simulink model "Simulink_Model_v12"  (R2020a)
settings: Solver=FixedStepAuto  StartTime=0.0  StopTime=150  FixedStep=1e-3  MaxStep=1e-2  RelTol=1e-3
PreLoadFcn:
  | addpath(genpath(pwd));
  | 
  | % ======================================================================= %
  | %% Physics Paramters
  | 
  | Physics_Param.gGravity        = 9.81;           % [m/s2]
  | Physics_Param.DAir            = 1.2;            % [kg/m3]
  | 
  | % ======================================================================= %
  | %% Tire Paramters
  | 
  | Tire_Param.muTire             = 1.75;           % [-]
  | 
  | Tire_Param.KTireLong          = 500;            % [rad^-1]
  | Tire_Param.KTireLat           = 1000;           % [rad^-1]
  | 
  | Tire_Param.CRollResistance    = 0.01;           % [-]
  | 
  | Tire_Param;
  | 
  | % ======================================================================= %
  | %% Motor Paramters
  | 
  | Motor_Param.PMotorMax         = 7.6*100;        % [W]
  | 
  | Motor_Param.nLimit            = 1000;           % [RPM]
  | 
  | Motor_Param.eDrivetrain       = 0.8*0.8*0.3;    % [-] %  \eta_i*\eta_d*correction_term
  | 
  | Motor_Param.rGearRatio1       = 3.3250;         % 84/48*38/20
  | Motor_Param.rGearRatio2       = 2.90;
  | 
  | % ======================================================================= %
  | %% Car Paramters
  | 
  | Car_Param.lCarWidth           = 0.2;            % [m]
  | Car_Param.hCarHeight          = 0.115;          % [m]
  | Car_Param.CCarDrag            = 0.3;            % [m]
  | 
  | Car_Param.lTrackWidth         = 0.165;          % [m]
  | Car_Param.lWheelbase          = 0.26;           % [m]
  | 
  | Car_Param.mWheel              = 0.03;           % [kg]
  | Car_Param.rWheel              = 0.03;           % [m]
  | Car_Param.IWheel              = 2.0760e-05;     % [kgm2] % 1/2*mWheel*(rWheel^2+0.022^2)
  | Car_Param.rWheelEffective     = 0.1885;         % [m]    % rWheel*2*pi
  | 
  | Car_Param.mCar                = 1.32;           % [kg]   % car mass
  | Car_Param.mCarSprung          = 1.198;          % [kg]   % mCar-4*mWheel
  | Car_Param.IzCar               = 0.0104;         % [kgm2] % 1/12*mCar*(lTrackWidth^2+lWheelbase^2)
  | 
  | Car_Param.hCenterGravity      = 0.02;           % [m]
  | 
  | Car_Param.hRollCenterF        = 0.01;           % [m]
  | Car_Param.hRollCenterR        = 0.01;           % [m]
  | 
  | Car_Param.KRollF              = 0.5;            % [N/m]
  | Car_Param.KRollR              = 0.5;            % [N/m]
  | 
  | Car_Param;
  | 
  | % ======================================================================= %
  | %% Track Select
  | 
  | % Track_Param.NTrack = 1;  % O-shape
  | % Track_Param.NTrack = 2;  % Oval-shape
  | 
  | Track_Param.NTrack = 5;  % Test track
  | % Track_Param.NTrack = 6;  % Test track
  | 
  | % Track_Param.NTrack = 10; % MCT
  | % Track_Param.NTrack = 11; % LMCC
  | 
  | % Track_Param.NTrack = 20; % AWS
  | 
  | run Track_Data\Track_Data.m
  | Track_Param.rTrajOpt = 0.009 %0.005;
  | 
  | % ======================================================================= %
  | %% Offline Trajectory Optimization
  | 
  | % run Trajectory_Optimizer.m
  | % Track_Param.xTrack=xTraj;
  | % Track_Param.yTrack=yTraj;
StopFcn:
  | Data1=out.CarPosition.Data;
  | 
  | figure(2)
  | cmap = colormap(jet);
  | s=scatter(Data1(:,1),Data1(:,2),0.1,Data1(:,4),'.');
  | c=colorbar;
  | ylabel(c,'v_{Car} (m/s)')
  | 
  | hold on
  | plot(Track_Param.xTrack,Track_Param.yTrack,'k')
  | plot(Track_Param.xRightSide',Track_Param.yRightSide','k--')
  | k=plot(Track_Param.xLeftSide' ,Track_Param.yLeftSide' ,'k--');
  | sf=plot(Track_Param.xStartLine,Track_Param.yStartLine,'k-.');
  | 
  | s.Annotation.LegendInformation.IconDisplayStyle = 'off';
  | k.Annotation.LegendInformation.IconDisplayStyle = 'off';
  | sf.Annotation.LegendInformation.IconDisplayStyle = 'off';
  | legend('Track centerline','Track limits')
  | axis off
  | text(0.5,-5,'S/F\rightarrow','HorizontalAlignment','center')
  | % title('Car position and velocity')
  | 
  | clear Data1 cmap s c k sf
libraries: simulink x8, dspfdesign x2
(part 1 of 2)
settings Model: Creator=arthu  LastModifiedBy=arthu
settings SolverCC: ZeroCrossAlgorithm=Adaptive
settings OptimizationCC: DefaultParameterBehavior=Inlined  EnhancedBackFolding=on  PassReuseOutputArgsAs=Individual arguments  ZeroExternalMemoryAtStartup=off  ZeroInternalMemoryAtStartup=off  OptimizeBlockOrder=speed  DifferentSizesBufferReuse=on  OptimizationCustomize=off  EfficientTunableParamExpr=on
settings DebuggingCC: ReadBeforeWriteMsg=DisableAll  WriteAfterWriteMsg=DisableAll  WriteAfterReadMsg=DisableAll  IgnoredZcDiagnostic=none  MultiTaskDSMMsg=none  ParameterTunabilityLossMsg=error
settings ModelReferenceCC: UpdateModelReferenceTargets=IfOutOfDate
settings SFSimCC: SFSimEcho=off  MATLABDynamicMemAlloc=off
settings RTWCC: SystemTargetFile=ert.tlc  TemplateMakefile=ert_default_tmf  BuildConfiguration=Faster Runs
settings CodeAppCC: ForceParamTrailComments=on  IgnoreCustomStorageClasses=off  OperatorAnnotations=on  SimulinkDataObjDesc=on  SFDataObjDesc=on  InsertBlockDesc=on
settings ERTTargetCC: TargetLangStandard=C99 (ISO)  GenerateSampleERTMain=on  InlinedParameterPlacement=NonHierarchical  ERTCustomFileTemplate=example_file_process.tlc

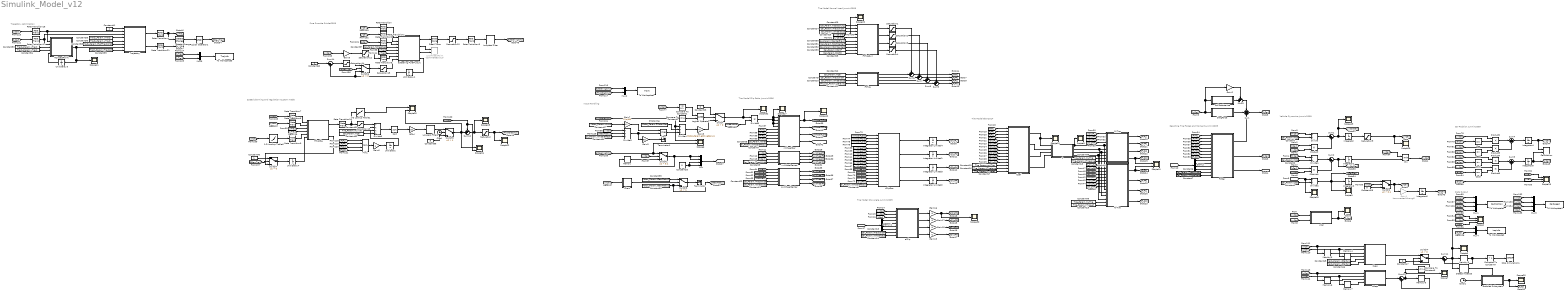
== system Simulink_Model_v12 ==
  note: Trajectory optimization
  note: Speed planning and regulation
      |
      | Custom made
  note: Pure Pursuite
      |
      | Snider2009
  note: Input Handling
  note: Tire Model
      | Slip Ratio
      |
      | Junmin2006
  note: Tire Model
      | Slip Angle
      |
      | Junmin2009
  note: Tire Model
      | Normal Load
      |
      | Junmin2009
  note: Tire Model
      |
      | Bian2014
  note: Resulting Tire Forces and Moment
      |
      | Junmin2009
  note: Vehicle Dynamics
      |
      | Junmin2009
  note: Data Output
  note: Car Position
      |
      | Junmin2009
  1-D Lookup Table1 : Lookup_n-D  NumberOfTableDimensions=1  BreakpointsForDimension1=[0,0.04,0.1,0.2,0.3,0.5]*1  Table=[20,10,9,6,5,4]  ExtrapMethod=Clip  InternalRulePriority=Speed  RndMeth=Simplest  InputSameDT=on
  1-D Lookup Table6 : Lookup_n-D  NumberOfTableDimensions=1  BreakpointsForDimension1=[7.5,10,15,20]  Table=[5,10,25,40]  ExtrapMethod=Clip  InternalRulePriority=Speed  OutDataTypeStr=Inherit: Inherit via back propagation  RndMeth=Simplest  InputSameDT=on
  CarPosition : simulink/Sinks/XY Graph  xmin=min(Track_Param.xTrack)-10  xmax=max(Track_Param.xTrack)+10  ymin=min(Track_Param.yTrack)-10  ymax=max(Track_Param.yTrack)+10  st=-1
  Chart : Stateflow chart  TreatAsAtomicUnit=on
  Clock : Clock
  Clock1 : Clock
  Coef : MATLAB Function  TreatAsAtomicUnit=on
  Compare To Constant1 : simulink/Logic and Bit Operations/Compare To Constant  relop=<=  const=0.1  OutDataTypeStr=boolean
  Compare To Constant2 : simulink/Logic and Bit Operations/Compare To Constant  relop=<=  const=0  OutDataTypeStr=boolean
  Compare To Constant3 : simulink/Logic and Bit Operations/Compare To Constant  relop=>=  const=1  OutDataTypeStr=boolean
  Compare To Constant4 : simulink/Logic and Bit Operations/Compare To Constant  relop=>  const=4  OutDataTypeStr=boolean
  Constant{,2,12,52} (4 alike) : Constant  Value=Car_Param.mCar
  Constant1 : Constant  Value=Car_Param.IzCar
  Constant{7,10,14,21,26,37} (6 alike) : Constant  Value=Car_Param.lWheelbase
  Constant11 : Constant  Value=Physics_Param.gGravity
  Constant{3,6,9,13,22,24} (6 alike) : Constant  Value=Car_Param.lTrackWidth
  Constant{15,48..49,51} (4 alike) : Constant  Value=Tire_Param.muTire
  Constant16 : Constant  Value=Tire_Param.KTireLong
  Constant17 : Constant  Value=Tire_Param.KTireLat
  Constant18 : Constant  Value=Tire_Param.KTireLong
  Constant19 : Constant  Value=Tire_Param.KTireLat
  Constant{20,23,28,47} (4 alike) : Constant  Value=0
  Constant25 : Constant  Value=Car_Param.KRollR
  Constant27 : Constant  Value=Motor_Param.nLimit  SampleTime=-1
  Constant29 : Constant  Value=Car_Param.mCarSprung
  Constant30 : Constant  Value=Car_Param.hCenterGravity
  Constant31 : Constant  Value=Car_Param.hRollCenterF
  Constant32 : Constant  Value=Car_Param.hRollCenterR
  Constant33 : Constant  Value=Car_Param.KRollF
  Constant34 : Constant  Value=Car_Param.rWheelEffective  SampleTime=-1
  Constant35 : Constant  Value=Motor_Param.rGearRatio2  SampleTime=-1
  Constant36 : Constant  Value=5
  Constant39 : Constant  Value=Track_Param.rTrajOpt
  Constant4 : Constant  Value=Car_Param.rWheelEffective  SampleTime=-1
  Constant40 : Constant
  Constant41 : Constant  OutDataTypeStr=boolean
  Constant45 : Constant  Value=Track_Param.xStartLine
  Constant46 : Constant  Value=Track_Param.yStartLine
  Constant5 : Constant  Value=Car_Param.IWheel  SampleTime=-1
  Constant50 : Constant  Value=Motor_Param.rGearRatio1  SampleTime=-1
  Constant53 : Constant  Value=Track_Param.xTrack
  Constant54 : Constant  Value=Track_Param.yTrack
  Constant55 : Constant  Value=Track_Param.xTrack
  Constant56 : Constant  Value=Track_Param.yTrack
  Constant58 : Constant  Value=Track_Param.lHalfTrackWidth
  Constant60 : Constant
  Constant8 : Constant  Value=Car_Param.rWheelEffective  SampleTime=-1
  Cos : Trigonometry  Operator=cos
  Cos1 : Trigonometry
  Cos2 : Trigonometry
  Cos3 : Trigonometry  Operator=cos
  Dead Zone : DeadZone  LowerValue=-0.5*pi/180  UpperValue=0.5*pi/180  SaturateOnIntegerOverflow=on
  Demux : Demux
  Demux1 : Demux
  Detect Change : simulink/Logic and Bit Operations/Detect Change  vinit=0  OutDataTypeStr=boolean
  Detect Increase : simulink/Logic and Bit Operations/Detect Increase  vinit=0.0  OutDataTypeStr=boolean
  Divide : Product  Inputs=*/
  Divide1 : Product  Inputs=*/
  Divide2 : Product  Inputs=*/
  Divide3 : Product  Inputs=**/
  Divide4 : Product  Inputs=**/
  Divide5 : Product  Inputs=/**/
  Divide6 : Product  Inputs=**
  DragForce : Subsystem
  Enabled Subsystem : Subsystem  TreatAsAtomicUnit=on
  FMCar : MATLAB Function  TreatAsAtomicUnit=on
  FxTire : MATLAB Function  TreatAsAtomicUnit=on
  FyTire : MATLAB Function  TreatAsAtomicUnit=on
  FzTire : MATLAB Function  TreatAsAtomicUnit=on
  FzTireDyn : MATLAB Function  TreatAsAtomicUnit=on
  Gain1 : Gain  Commented=through  Gain=1/10
  Gain{16..19} (4 alike) : Gain  Gain=-1
  Gain2 : Gain  Gain=0.05
  Gain3 : Gain  Gain=60
  Gain5 : Gain  Gain=0.25
  Gain6 : Gain  Gain=4
  Gain7 : Gain  Gain=2*pi/60
  Gain8 : Gain  Gain=Motor_Param.eDrivetrain/4
  Integrator{,2,4..6} (5 alike) : Integrator
  Integrator Limited{1..4} (4 alike) : Integrator  LimitOutput=on  UpperSaturationLimit=10*pi/180  LowerSaturationLimit=-10*pi/180
  Integrator1 : Integrator  LimitOutput=on  UpperSaturationLimit=1  LowerSaturationLimit=-1
  Logical Operator : Logic  AllPortsSameDT=off  OutDataTypeStr=boolean
  Logical Operator1 : Logic  Inputs=1  AllPortsSameDT=off  OutDataTypeStr=boolean
  LookAheadPoint : simulink/Sinks/XY Graph  Commented=on  xmin=min(Track_Param.xTrack)-10  xmax=max(Track_Param.xTrack)+10  ymin=min(Track_Param.yTrack)-10  ymax=max(Track_Param.yTrack)+10  st=-1
  Lowpass Filter : dspfdesign/Lowpass Filter  FilterType=FIR  DesignForMinimumOrder=on  FilterOrder=50  PassbandFrequency=50  StopbandFrequency=100  PassbandRipple=0.1  StopbandAttenuation=50  InheritSampleRate=off  SampleRate=1000  SimulateUsing=Interpreted execution  roundingMode=Floor  coeffsDataTypeStr=fixdt(1,16)
  Lowpass Filter1 : dspfdesign/Lowpass Filter  FilterType=FIR  DesignForMinimumOrder=on  FilterOrder=50  PassbandFrequency=2  StopbandFrequency=10  PassbandRipple=0.1  StopbandAttenuation=50  InheritSampleRate=off  SampleRate=1000  SimulateUsing=Interpreted execution  roundingMode=Floor  coeffsDataTypeStr=fixdt(1,16)
  Max : MinMax  Function=max  Inputs=2
  Memory{,3..4,6..8} (6 alike) : Memory
  Memory5 : Memory  InitialCondition=1
  Min : MinMax  Inputs=2
  Min1 : MinMax  Inputs=4
  Mux : Mux
  Mux1 : Mux
  Mux2 : Mux  Inputs=2
  Mux3 : Mux  Inputs=2
  Mux4 : Mux  Inputs=2
  Mux5 : Mux
  NClosestPoint : MATLAB Function  TreatAsAtomicUnit=on
  NLap : MATLAB Function  TreatAsAtomicUnit=on
  PMotorMax : Constant  Value=Motor_Param.PMotorMax  SampleTime=-1
  Product{,1..5} (6 alike) : Product
  Rate Transition{,1..2,4..5,7..9,21} (9 alike) : RateTransition  OutPortSampleTime=0.01
  Rate Transition10 : RateTransition  OutPortSampleTime=0.001
  Rate Transition16 : RateTransition  OutPortSampleTime=0.1
  Rate Transition17 : RateTransition  OutPortSampleTime=0.1
  Rate Transition3 : RateTransition  OutPortSampleTime=0.001
  RollResistance : Subsystem
  Saturation : Saturate  UpperLimit=1  LowerLimit=-1
  Saturation{1..4} (4 alike) : Saturate  UpperLimit=Car_Param.mCar*Physics_Param.gGravity  LowerLimit=-Car_Param.mCar*Physics_Param.gGravity/4
  Saturation10 : Saturate  UpperLimit=26*pi/180  LowerLimit=-26*pi/180
  Saturation12 : Saturate  UpperLimit=5  LowerLimit=1
  Saturation13 : Saturate  UpperLimit=inf  LowerLimit=0.01
  Saturation14 : Saturate  UpperLimit=100  LowerLimit=1
  Saturation15 : Saturate  UpperLimit=100  LowerLimit=1
  Saturation9 : Saturate  UpperLimit=inf  LowerLimit=0
  Scope{,3,5,7,9,11..13,16..17,19..20,22,25,28..30,32} (18 alike) : Scope
  Scope{6,10,26,34} (4 alike) : Scope  NumInputPorts=2
  Scope15 : Scope  NumInputPorts=3
  Scope2 : Scope  NumInputPorts=3
  Sqrt : Sqrt  SaturateOnIntegerOverflow=on
  Stop Simulation1 : Stop
  Sum : Sum  Inputs=--+
  Sum{1,5,11,13} (4 alike) : Sum  Inputs=|++
  Sum12 : Sum  Inputs=-+|
  Sum14 : Sum  Inputs=|-+
  Sum2 : Sum  Inputs=|+-
  Sum{3,6..9} (5 alike) : Sum  Inputs=++|
  Sum4 : Sum  Inputs=|+-
  Switch{,4,6..7} (4 alike) : Switch  Criteria=u2 > Threshold
  Switch1 : Switch  Criteria=u2 > Threshold  Threshold=0.1
  Switch2 : Switch  Criteria=u2 > Threshold  Threshold=0.1
  Switch5 : Switch  Criteria=u2 > Threshold  Threshold=1
  Switch8 : Switch  Criteria=u2 > Threshold  Threshold=1
  Terminator : Terminator
  Terminator1 : Terminator
  To Workspace : ToWorkspace  VariableName=CarPosition  SaveFormat=Timeseries  SampleTime=-1
  To Workspace1 : ToWorkspace  VariableName=Input  SaveFormat=Timeseries  SampleTime=-1
  To Workspace2 : ToWorkspace  VariableName=LapInfo  SaveFormat=Timeseries  SampleTime=-1
  To Workspace3 : ToWorkspace  VariableName=TrajInfo  SaveFormat=Timeseries  SampleTime=-1
  To Workspace4 : ToWorkspace  VariableName=CarSpeed  SaveFormat=Timeseries  SampleTime=-1
  Trajectory : MATLAB Function  TreatAsAtomicUnit=on
  Unit Delay : UnitDelay  SampleTime=0.001  HasFrameUpgradeWarning=on
  Unit Delay1 : UnitDelay  InitialCondition=1  SampleTime=-1  HasFrameUpgradeWarning=on
  Unit Delay3 : UnitDelay  InitialCondition=1  SampleTime=-1  HasFrameUpgradeWarning=on
  Unit Delay4 : UnitDelay  InitialCondition=1  SampleTime=-1  HasFrameUpgradeWarning=on
  \eta_v : Gain  Gain=0.8
  aSlip : MATLAB Function  TreatAsAtomicUnit=on
  aSteering PurePursuit : MATLAB Function  TreatAsAtomicUnit=on
  axWheelCenter : MATLAB Function  TreatAsAtomicUnit=on
  f : MATLAB Function  TreatAsAtomicUnit=on
  nWheelDer : MATLAB Function  TreatAsAtomicUnit=on
  rSlipDer : MATLAB Function  TreatAsAtomicUnit=on
  rThrottle : MATLAB Function  TreatAsAtomicUnit=on
  sStep : MATLAB Function  TreatAsAtomicUnit=on
  vCar : MATLAB Function  TreatAsAtomicUnit=on
  vxWheelCenter : MATLAB Function  TreatAsAtomicUnit=on
  wires:
  [FxCar] -> Divide/1
  Constant/1 -> Divide/2
  Divide/1 -> Sum1/1
  [rCar] -> Product/1
  [vyCar] -> Product/2
  Product/1 -> Sum1/2
  Sum1/1 -> Scope19/1, [vxCarDer], Integrator/1
  Integrator/1 -> Saturation9/1
  [vxCar] -> Product1/2
  [rCar] -> Product1/1
  Constant2/1 -> Divide1/2
  [FyCar] -> Divide1/1
  Divide1/1 -> Sum2/1
  Product1/1 -> Sum2/2
  Sum2/1 -> [vyCarDer], Integrator1/1
  Demux1/1 -> aSlip/4(aSteerFL)
  FMCar/1(FxCar) -> Sum/3
  Sum/1 -> [FxCar]
  DragForce/1(FDrag) -> Sum/2
  [vxCar] -> vCar/1(vxCar)
  [vyCar] -> vCar/2(vyCar)
  vCar/1(vCar) -> [vCar], Scope/1  "vCar"
  [vCar] -> Gain2/1, RollResistance/1(vCar), DragForce/1(vCar)
  [aSteer] -> Demux/1
  Demux/1 -> FMCar/9(aSteerFL)
  Demux/4 -> FMCar/12(aSteerRR)
  Demux/2 -> FMCar/10(aSteerFR)
  Demux/3 -> FMCar/11(aSteerRL)
  Constant6/1 -> FMCar/13(lTrackWidth)
  Constant7/1 -> FMCar/14(lWheelbase)
  Constant3/1 -> vxWheelCenter/4(lTrackWidth)
  [rCar] -> vxWheelCenter/3(rCar)
  [vyCar] -> vxWheelCenter/2(vyCar)
  [vxCar] -> vxWheelCenter/1(vxCar)
  Constant8/1 -> rSlipDer/17(rWheelEffective)
  FzTire/1(FzFL) -> Sum6/2  "FzFL"
  FzTire/2(FzFR) -> Sum7/2  "FzFR"
  FzTire/3(FzRL) -> Sum8/2  "FzRL"
  FzTire/4(FzRR) -> Sum9/2  "FzRR"
  Constant12/1 -> FzTire/1(mCar)
  Constant9/1 -> FzTire/2(lTrackWidth)
  Constant10/1 -> FzTire/3(lWheelbase)
  Constant11/1 -> FzTire/4(gGravity)
  [rCar] -> aSlip/3(rCar)
  [vxCar] -> aSlip/1(VxCar)
  [vyCar] -> aSlip/2(VyCar)
  [aSteer] -> Demux1/1
  Demux1/2 -> aSlip/5(aSteerFR)
  Demux1/3 -> aSlip/6(aSteerRL)
  Demux1/4 -> aSlip/7(aSteerRR)
  Constant13/1 -> aSlip/8(lTrackWidth)
  Constant14/1 -> aSlip/9(lWheelbase)
  [FzFL] -> Coef/1(FzFL)
  [FzFR] -> Coef/2(FzFR)
  [FzRL] -> Coef/3(FzRL)
  [FzRR] -> Coef/4(FzRR)
  aSlip/1(aSlipFL) -> Gain16/1  "aSlipFL"
  aSlip/2(aSlipFR) -> Gain17/1  "aSlipFR"
  aSlip/3(aSlipRL) -> Gain18/1  "aSlipRL"
  aSlip/4(aSlipRR) -> Gain19/1  "aSlipRR"
  Constant15/1 -> Coef/13(muTire)
  Constant16/1 -> Coef/14(KTireLong)
  Constant17/1 -> Coef/15(KTireLat)
  [rSlipFR] -> Coef/6(rSlipFR)
  [rSlipFL] -> Coef/5(rSlipFL)
  [rSlipRL] -> Coef/7(rSlipRL)
  [rSlipRR] -> Coef/8(rSlipRR)
  [aSlipFL] -> Coef/9(aSlipFL)
  [aSlipFR] -> Coef/10(aSlipFR)
  [aSlipRL] -> Coef/11(aSlipRL)
  [aSlipRR] -> Coef/12(aSlipRR)
  Coef/1(CoefFL) -> Scope13/1, f/1(CoefFL)
  Coef/2(CoefFR) -> f/2(CoefFR)
  Coef/3(CoefRL) -> f/3(CoefRL)
  Coef/4(CoefRR) -> f/4(CoefRR)
  f/1(fCoefFL) -> FyTire/9(fCoefFL), FxTire/5(fCoefFL), Scope9/1
  f/2(fCoefFR) -> FyTire/10(fCoefFR), FxTire/6(fCoefFR)
  f/3(fCoefRL) -> FyTire/11(fCoefRL), FxTire/7(fCoefRL)
  f/4(fCoefRR) -> FxTire/8(fCoefRR), FyTire/12(fCoefRR)
  [rSlipFL] -> FxTire/1(rSlipFL)
  [rSlipFR] -> FxTire/2(rSlipFR)
  [rSlipRL] -> FxTire/3(rSlipRL)
  [rSlipRR] -> FxTire/4(rSlipRR)
  Constant18/1 -> FxTire/10(KTireLong)
  [FxFL] -> FMCar/1(FxFL)
  [FxFR] -> FMCar/2(FxFR)
  [FxRL] -> FMCar/3(FxRL)
  [FxRR] -> FMCar/4(FxRR)
  [rSlipFL] -> FyTire/5(rSlipFL)
  [rSlipFR] -> FyTire/6(rSlipFR)
  [rSlipRL] -> FyTire/7(rSlipRL)
  [rSlipRR] -> FyTire/8(rSlipRR)
  Constant19/1 -> FyTire/14(KTireLat)
  [aSlipFL] -> FyTire/1(aSlipFL)
  [aSlipFR] -> FyTire/2(aSlipFR)
  [aSlipRL] -> FyTire/3(aSlipRL)
  [aSlipRR] -> FyTire/4(aSlipRR)
  FyTire/1(FyFL) -> Scope10/2, [FyFL]
  FyTire/2(FyFR) -> [FyFR]
  FyTire/3(FyRL) -> [FyRL]
  FyTire/4(FyRR) -> [FyRR]
  [FyFL] -> FMCar/5(FyFL)
  [FyFR] -> FMCar/6(FyFR)
  [FyRL] -> FMCar/7(FyRL)
  [FyRR] -> FMCar/8(FyRR)
  Gain17/1 -> [aSlipFR]
  Gain18/1 -> [aSlipRL]
  Gain19/1 -> [aSlipRR]
  Mux/1 -> [aSteer]
  FxTire/1(FxFL) -> [FxFL]
  FxTire/2(FxFR) -> [FxFR]
  FxTire/3(FxRL) -> [FxRL]
  FxTire/4(FxRR) -> [FxRR], Scope10/1
  [vxCar] -> Scope2/1  "vxCar"
  [vyCar] -> Scope2/2  "vyCar"
  [rCar] -> Scope2/3  "rCar"
  Integrator Limited4/1 -> [rSlipFL]
  Integrator Limited1/1 -> [rSlipFR]
  Integrator Limited3/1 -> [rSlipRL]
  Integrator Limited2/1 -> [rSlipRR]
  Constant20/1 -> Mux/3, Mux/4
  Switch1/1 -> Memory/1, Mux/2, Mux/1
  vxWheelCenter/1(vxWheelFL) -> [vxWheelFL]
  vxWheelCenter/2(vxWheelFR) -> [vxWheelFR]
  vxWheelCenter/3(vxWheelRL) -> [vxWheelRL]
  vxWheelCenter/4(vxWheelRR) -> [vxWheelRR]
  [vxWheelRR] -> rSlipDer/8(vxWheelRR)
  [vxWheelRL] -> rSlipDer/7(vxWheelRL)
  [vxWheelFR] -> rSlipDer/6(vxWheelFR)
  [vxWheelFL] -> rSlipDer/5(vxWheelFL)
  [FxFL] -> nWheelDer/5(FxFL)
  [FxFR] -> nWheelDer/6(FxFR)
  [FxRL] -> nWheelDer/7(FxRL)
  [FxRR] -> nWheelDer/8(FxRR)
  Constant4/1 -> nWheelDer/10(rWheelEffective)
  Constant5/1 -> nWheelDer/9(IWheel)
  [rCar] -> axWheelCenter/1(rCar)
  [vxCarDer] -> axWheelCenter/2(vxCarDer)
  [vyCarDer] -> axWheelCenter/3(vyCarDer)
  [rCarDer] -> axWheelCenter/4(rCarDer)
  Constant21/1 -> axWheelCenter/6(lWheelbase)
  Constant22/1 -> axWheelCenter/5(lTrackWidth)
  axWheelCenter/1(axWheelFL) -> [axWheelFL]
  axWheelCenter/2(axWheelFR) -> [axWheelFR]
  axWheelCenter/3(axWheelRL) -> [axWheelRL]
  axWheelCenter/4(axWheelRR) -> [axWheelRR]
  [axWheelFR] -> rSlipDer/10(axWheelFR)
  [axWheelFL] -> rSlipDer/9(axWheelFL)
  [axWheelRL] -> rSlipDer/11(axWheelRL)
  [axWheelRR] -> rSlipDer/12(axWheelRR)
  [rSlipFL] -> rSlipDer/13(rSlipFL)
  [rSlipFR] -> rSlipDer/14(rSlipFR)
  [rSlipRL] -> rSlipDer/15(rSlipRL)
  [rSlipRR] -> rSlipDer/16(rSlipRR)
  Divide6/1 -> nWheelDer/1(MWheelFL), Scope17/1, nWheelDer/2(MWheelFR), nWheelDer/3(MWheelRL), nWheelDer/4(MWheelRR)  "MWheel"
  nWheelDer/1(nWheelFLDer) -> Scope12/1, [nWheelFLDer]
  nWheelDer/2(nWheelFRDer) -> [nWheelFRDer]
  nWheelDer/4(nWheelRRDer) -> [nWheelRRDer]
  nWheelDer/3(nWheelRLDer) -> [nWheelRLDer]
  [nWheelFLDer] -> rSlipDer/1(nWheelFLDer)
  [nWheelFRDer] -> rSlipDer/2(nWheelFRDer)
  [nWheelRLDer] -> rSlipDer/3(nWheelRLDer)
  [nWheelRRDer] -> rSlipDer/4(nWheelRRDer)
  Logical Operator/1 -> Switch/2
  [vCar] -> Compare To Constant1/1
  Compare To Constant1/1 -> Logical Operator/1
  Constant23/1 -> Switch/1
  [MzCar] -> Scope16/1, Divide2/1
  Sum4/1 -> Integrator4/1
  [vyCar] -> Product5/1
  Product5/1 -> Sum5/2
  Cos2/1 -> Product4/2
  Cos3/1 -> Product5/2
  [vxCar] -> Product4/1
  Product4/1 -> Sum5/1
  [aCar] -> Scope15/3  "aCar"
  [vyCar] -> Product3/1
  Cos1/1 -> Product3/2
  [aCar] -> Cos2/1
  Sum5/1 -> Integrator5/1
  [vxCar] -> Product2/1
  Cos/1 -> Product2/2
  [aCar] -> Cos3/1
  [aCar] -> Cos/1
  Product3/1 -> Sum4/2
  [aCar] -> Cos1/1
  Product2/1 -> Sum4/1
  Integrator6/1 -> [aCar]
  Integrator4/1 -> CarPosition/1, [xCar]  "xCar"
  Switch2/1 -> Gain1/1, [rCar]
  FMCar/2(FyCar) -> [FyCar]
  [yCar] -> Mux1/2
  [xCar] -> Mux1/1
  Mux1/1 -> To Workspace/1
  [vCar] -> Mux1/4
  Constant26/1 -> FzTireDyn/3(lWheelbase)
  Constant33/1 -> FzTireDyn/9(KRollF)
  Constant29/1 -> FzTireDyn/1(mCarSprung)
  Constant25/1 -> FzTireDyn/10(KRollR)
  Constant30/1 -> FzTireDyn/6(hCentrerGravity)
  Constant24/1 -> FzTireDyn/2(lTrackWidth)
  Constant32/1 -> FzTireDyn/8(hRollCenterR)
  Constant31/1 -> FzTireDyn/7(hRollCenterF)
  [vxCarDer] -> Scope20/1, FzTireDyn/4(axCar)
  [vyCarDer] -> FzTireDyn/5(ayCar)
  Sum9/1 -> [FzRR]  "FzRR"
  Sum8/1 -> [FzRL]  "FzRL"
  Sum7/1 -> [FzFR]  "FzFR"
  Sum6/1 -> [FzFL]  "FzFL"
  Integrator5/1 -> CarPosition/2, [yCar]  "yCar"
  [xCar] -> Scope15/1
  [yCar] -> Scope15/2
  FzTireDyn/4(FzRR) -> Saturation4/1
  FzTireDyn/3(FzRL) -> Saturation3/1
  FzTireDyn/2(FzFR) -> Saturation2/1
  FzTireDyn/1(FzFL) -> Saturation1/1
  Sum3/1 -> Sum/1
  [vxCar] -> Min/1
  Constant28/1 -> Switch2/3
  [vxCar] -> Switch2/2
  Compare To Constant2/1 -> Logical Operator/2
  [vxCar] -> Divide3/1
  Constant34/1 -> Divide3/3
  Divide3/1 -> Gain3/1, Max/2  "nMotor tr/s"
  PMotorMax/1 -> Divide4/2
  Divide4/1 -> Gain8/1
  Min/1 -> [vyCar]
  Constant27/1 -> Gain7/1
  Max/1 -> Divide4/3
  [vxCar] -> Switch1/2
  Memory/1 -> Switch1/3
  Constant1/1 -> Divide2/2
  Saturation9/1 -> Scope29/1, [vxCar]
  Integrator1/1 -> Min/2
  Integrator2/1 -> Switch2/1
  Gain1/1 -> Integrator6/1
  Divide2/1 -> [rCarDer], Scope3/1, Integrator2/1
  RollResistance/1(FRollResistance) -> Sum3/2
  Gain2/1 -> Sum3/1
  [xCar] -> Rate Transition/1
  [yCar] -> Rate Transition1/1
  [aCar] -> Rate Transition2/1
  Constant37/1 -> aSteering PurePursuit/4(lWheelBase)
  Dead Zone/1 -> Saturation10/1
  Rate Transition/1 -> aSteering PurePursuit/1(xCar)
  Rate Transition1/1 -> aSteering PurePursuit/2(yCar)
  Rate Transition2/1 -> aSteering PurePursuit/3(aCar)
  aSteering PurePursuit/3(yLookAheadPoint) -> LookAheadPoint/2
  aSteering PurePursuit/2(xLookAheadPoint) -> LookAheadPoint/1
  [rThrottleCmd] -> Scope6/1, Divide4/1, Compare To Constant2/1
  [aSteeringCmd] -> Scope6/2, Switch1/1
  [vxCar] -> Scope34/2, Sum12/1
  Rate Transition5/1 -> aSteering PurePursuit/7(sLookAhead)
  Rate Transition8/1 -> rThrottle/2(yCar)
  Rate Transition7/1 -> rThrottle/1(xCar)
  [yCar] -> Rate Transition8/1
  [xCar] -> Rate Transition7/1
  rThrottle/1(KMax) -> Rate Transition10/1
  [vxCar] -> 1-D Lookup Table6/1
  Rate Transition9/1 -> rThrottle/5(sAnticipation)
  Saturation1/1 -> Sum6/1
  Saturation2/1 -> Sum7/1
  Saturation3/1 -> Sum8/1
  Saturation4/1 -> Sum9/1
  Saturation/1 -> Scope22/1, [rThrottleCmd]
  \eta_v/1 -> Lowpass Filter1/1
  Constant45/1 -> NLap/5(xStartLine)
  Constant46/1 -> NLap/6(yStartLine)
  [xCar] -> Memory3/1, NLap/1(xCar)
  [yCar] -> Memory4/1, NLap/2(yCar)
  Memory3/1 -> NLap/3(xCarPrev)
  Memory4/1 -> NLap/4(yCarPrev)
  NLap/1(BNewLap) -> Switch4/1
  Sum11/1 -> Mux4/1, Scope5/1, Detect Increase/1, Memory5/1  "NLap"
  Memory5/1 -> Compare To Constant4/1, Sum11/2
  Memory6/1 -> sStep/3(xCarPrev)
  Memory7/1 -> sStep/4(yCarPrev)
  [yCar] -> Memory7/1, sStep/2(yCar)
  [xCar] -> Memory6/1, sStep/1(xCar)
  Memory8/1 -> Sum13/2
  Sum13/1 -> Memory8/1, Scope7/1, Compare To Constant3/1  "sCovered"
  sStep/1(sStep) -> Sum13/1
  Compare To Constant3/1 -> Switch4/2
  Switch4/1 -> Sum11/1
  Constant47/1 -> Switch4/3
  Lowpass Filter/1 -> [aSteeringCmd]
  aSteering PurePursuit/1(aSteeringCmd) -> Dead Zone/1
  [aSteeringCmd] -> Mux2/1
  Mux2/1 -> To Workspace1/1
  [rThrottleCmd] -> Mux2/2
  [FzFL] -> Min1/1
  [FzFR] -> Min1/2
  [FzRL] -> Min1/3
  [FzRR] -> Min1/4
  Divide5/1 -> Sqrt/1
  Sqrt/1 -> \eta_v/1
  Constant51/1 -> Divide5/3
  Constant52/1 -> Divide5/4
  Saturation13/1 -> Divide5/1
  Min1/1 -> Gain6/1
  Gain6/1 -> Unit Delay/1
  Unit Delay/1 -> Divide5/2
  Gain7/1 -> Max/1
  Gain8/1 -> Switch/3
  Saturation10/1 -> Rate Transition3/1
  Rate Transition3/1 -> Lowpass Filter/1
  Clock/1 -> Switch5/2
  Lowpass Filter1/1 -> Switch5/1
  Constant36/1 -> Switch5/3
  Rate Transition10/1 -> Saturation13/1, 1-D Lookup Table1/1
  1-D Lookup Table1/1 -> Scope26/1
  Constant53/1 -> NClosestPoint/3(xTrack)
  Constant54/1 -> NClosestPoint/4(yTrack)
  [yCar] -> Rate Transition17/1
  [xCar] -> Rate Transition16/1
  Unit Delay3/1 -> NClosestPoint/5(NClosestPointPrev)
  Constant55/1 -> Trajectory/4(xTrack)
  Constant56/1 -> Trajectory/5(yTrack)
  NClosestPoint/1(NClosestPoint) -> Trajectory/7(NClosestPoint), Scope11/1, Unit Delay3/1
  Rate Transition17/1 -> NClosestPoint/2(yCar), Trajectory/3(yCar)
  Rate Transition16/1 -> NClosestPoint/1(xCar), Trajectory/2(xCar)
  Constant58/1 -> Trajectory/6(lHalfTrackWidth)
  Constant39/1 -> Trajectory/8(rTrajOpt)
  aSteering PurePursuit/4(NLookAheadOpt) -> Unit Delay1/1
  Switch6/1 -> Saturation15/1
  Saturation14/1 -> Switch6/1
  [xTraj] -> aSteering PurePursuit/5(xTrack)
  [xTraj] -> rThrottle/3(xTrack)
  Rate Transition21/1 -> [yTraj]
  [yTraj] -> aSteering PurePursuit/6(yTrack)
  [yTraj] -> rThrottle/4(yTrack)
  Detect Change/1 -> Logical Operator1/1
  Constant40/1 -> Switch7/1
  Switch7/1 -> Unit Delay4/1
  Rate Transition4/1 -> Detect Change/1, [xTraj]
  Saturation15/1 -> aSteering PurePursuit/8(NLookAheadPrev)
  Unit Delay4/1 -> rThrottle/6(NClosestPointPrev)
  rThrottle/3(NClosestPoint) -> Switch7/3
  Constant41/1 -> Trajectory/1(BOpt)
  Compare To Constant4/1 -> Stop Simulation1/1
  Mux3/1 -> To Workspace3/1
  [xTraj] -> Mux3/1
  [yTraj] -> Mux3/2
  [aCar] -> Mux1/3
  Detect Increase/1 -> Enabled Subsystem/Enable
  Clock1/1 -> Enabled Subsystem/1(In1)
  Enabled Subsystem/1(Out1) -> [tLap], Scope25/1
  Constant35/1 -> Switch8/1
  [vCar] -> Chart/1(vCar)
  Chart/1(Gear) -> Switch8/2
  1-D Lookup Table6/1 -> Rate Transition9/1
  rSlipDer/1(rSlipFLDer) -> Integrator Limited4/1
  rSlipDer/2(rSlipFRDer) -> Integrator Limited1/1
  rSlipDer/3(rSlipRLDer) -> Integrator Limited3/1
  rSlipDer/4(rSlipRRDer) -> Integrator Limited2/1
  Mux4/1 -> To Workspace2/1
  [tLap] -> Mux4/2
  [rGearRatio] -> Divide3/2
  Switch/1 -> Scope32/1, Divide6/1  "MMotor"
  [rGearRatio] -> Divide6/2
  Constant50/1 -> [rGearRatio], Switch8/3
  Gain3/1 -> Terminator1/1  "nMotor RPM"
  Constant48/1 -> FxTire/9(muTire)
  Constant49/1 -> FyTire/13(muTire)
  Mux5/1 -> To Workspace4/1
  [vxCar] -> Mux5/1
  [vyCar] -> Mux5/2
  [vCar] -> Mux5/3
  [rCar] -> Mux5/4
  Logical Operator1/1 -> [BNewTraj]
  [BNewTraj] -> Switch6/2
  [BNewTraj] -> Switch7/2
  Trajectory/1(xTraj) -> Rate Transition4/1
  Trajectory/2(yTraj) -> Rate Transition21/1
  Constant60/1 -> Sum14/1
  Unit Delay1/1 -> Sum14/2, Switch6/3
  [vxCar] -> Gain5/1
  Gain5/1 -> Saturation12/1
  Saturation12/1 -> Rate Transition5/1
  Switch5/1 -> Scope34/1, Sum12/2, Scope26/2
  FMCar/3(MzCar) -> [MzCar]
  Gain16/1 -> Scope30/1, [aSlipFL]
  Sum14/1 -> Saturation14/1
  Sum12/1 -> Scope28/1, Saturation/1
  Switch8/1 -> Terminator/1

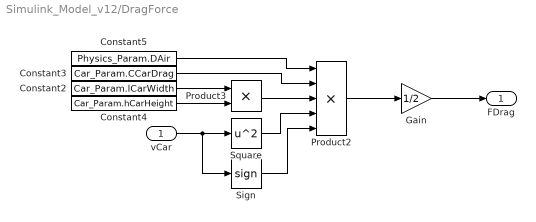
== system Simulink_Model_v12/DragForce ==
  vCar : Inport
  Constant2 : Constant  Value=Car_Param.lCarWidth
  Constant3 : Constant  Value=Car_Param.CCarDrag
  Constant4 : Constant  Value=Car_Param.hCarHeight
  Constant5 : Constant  Value=Physics_Param.DAir
  Gain : Gain  Gain=1/2
  Product2 : Product  Inputs=5
  Product3 : Product
  Sign : Signum
  Square : Math  Operator=square  SaturateOnIntegerOverflow=on
  FDrag : Outport
  wires:
  Gain/1 -> FDrag/1
  Constant3/1 -> Product2/2
  Constant5/1 -> Product2/1
  Square/1 -> Product2/4
  Constant2/1 -> Product3/1
  Product2/1 -> Gain/1
  Product3/1 -> Product2/3
  Constant4/1 -> Product3/2
  vCar/1 -> Sign/1, Square/1
  Sign/1 -> Product2/5

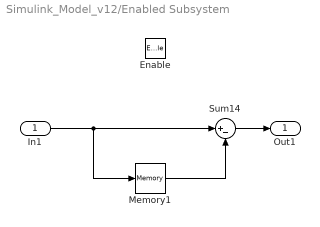
== system Simulink_Model_v12/Enabled Subsystem ==
  In1 : Inport
  Enable : EnablePort
  Memory1 : Memory
  Sum14 : Sum  Inputs=|+-
  Out1 : Outport
  wires:
  In1/1 -> Sum14/1, Memory1/1
  Sum14/1 -> Out1/1
  Memory1/1 -> Sum14/2

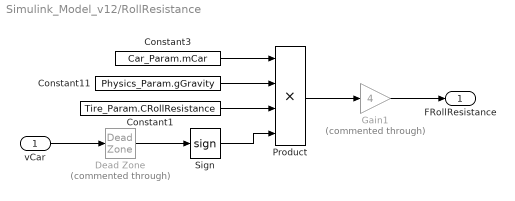
== system Simulink_Model_v12/RollResistance ==
  vCar : Inport
  Constant1 : Constant  Value=Tire_Param.CRollResistance
  Constant11 : Constant  Value=Physics_Param.gGravity
  Constant3 : Constant  Value=Car_Param.mCar
  Dead Zone : DeadZone  Commented=through  LowerValue=-1  UpperValue=1  SaturateOnIntegerOverflow=on
  Gain1 : Gain  Commented=through  Gain=4
  Product : Product  Inputs=4
  Sign : Signum
  FRollResistance : Outport
  wires:
  Product/1 -> Gain1/1
  Constant11/1 -> Product/2
  Constant3/1 -> Product/1
  Constant1/1 -> Product/3
  vCar/1 -> Dead Zone/1
  Dead Zone/1 -> Sign/1
  Sign/1 -> Product/4
  Gain1/1 -> FRollResistance/1

== matlab function Simulink_Model_v12/FzTireDyn ==
  data: FzFL output; mCarSprung input; lTrackWidth input; lWheelbase input; axCar input; ayCar input; hCentrerGravity input; hRollCenterF input; hRollCenterR input; KRollF input; KRollR input; FzFR output; FzRL output; FzRR output
function [FzFL,FzFR,FzRL,FzRR]...
         = FzTireDyn(mCarSprung,lTrackWidth,lWheelbase,...
                     axCar,ayCar,...
                     hCentrerGravity,hRollCenterF,hRollCenterR,KRollF,KRollR)

FzFL=-mCarSprung*axCar*hCentrerGravity/lWheelbase...
     -mCarSprung*ayCar*hRollCenterF*KRollF/lTrackWidth;

FzFR=-mCarSprung*axCar*hCentrerGravity/lWheelbase...
     +mCarSprung*ayCar*hRollCenterF*KRollF/lTrackWidth;

FzRL=+mCarSprung*axCar*hCentrerGravity/lWheelbase...
     -mCarSprung*ayCar*hRollCenterR*KRollR/lTrackWidth;

FzRR=+mCarSprung*axCar*hCentrerGravity/lWheelbase...
     +mCarSprung*ayCar*hRollCenterR*KRollR/lTrackWidth;

end

== matlab function Simulink_Model_v12/FzTire ==
  data: mCar input; FzFL output; lTrackWidth input; lWheelbase input; gGravity input; FzFR output; FzRL output; FzRR output
function [FzFL,FzFR,FzRL,FzRR]...
         = FzTire(mCar,...
                  lTrackWidth,lWheelbase,...
                  gGravity)

FzFL=mCar*gGravity*(lWheelbase/2)/(2*lWheelbase);

FzFR=mCar*gGravity*(lWheelbase/2)/(2*lWheelbase);

FzRL=mCar*gGravity*(lWheelbase/2)/(2*lWheelbase);

FzRR=mCar*gGravity*(lWheelbase/2)/(2*lWheelbase);

end

== matlab function Simulink_Model_v12/aSlip ==
  data: VxCar input; aSlipFL output; aSlipFR output; aSlipRL output; aSlipRR output; VyCar input; rCar input; aSteerFL input; aSteerFR input; aSteerRL input; aSteerRR input; lTrackWidth input; lWheelbase input
function [aSlipFL,aSlipFR,aSlipRL,aSlipRR]...
         = aSlip(VxCar,VyCar,rCar,...
                 aSteerFL,aSteerFR,aSteerRL,aSteerRR,...
                 lTrackWidth,lWheelbase)

if abs(VxCar-rCar*lTrackWidth/2)<=1
    aSlipFL=-aSteerFL+atan((VyCar+rCar*lWheelbase/2));
    
    aSlipRL=-aSteerRL+atan((VyCar-rCar*lWheelbase/2));
else
    aSlipFL=-aSteerFL+atan((VyCar+rCar*lWheelbase/2)/(VxCar-rCar*lTrackWidth/2));
    
    aSlipRL=-aSteerRL+atan((VyCar-rCar*lWheelbase/2)/(VxCar-rCar*lTrackWidth/2));
end

if abs(VxCar+rCar*lTrackWidth/2)<=1
    aSlipFR=-aSteerFR+atan((VyCar+rCar*lWheelbase/2));
    
    aSlipRR=-aSteerRR+atan((VyCar-rCar*lWheelbase/2));
else
    aSlipFR=-aSteerFR+atan((VyCar+rCar*lWheelbase/2)/(VxCar+rCar*lTrackWidth/2));
    
    aSlipRR=-aSteerRR+atan((VyCar-rCar*lWheelbase/2)/(VxCar+rCar*lTrackWidth/2));
end

end

% ======================================================================= %

% if abs(VxCar)<=1
%     aSlipFL=-aSteerFL+atan((VyCar+rCar*lWheelbase/2));
%     
%     aSlipFR=-aSteerFR+atan((VyCar+rCar*lWheelbase/2));
%     
%     aSlipRL=-aSteerRL+atan((VyCar-rCar*lWheelbase/2));
%     
%     aSlipRR=-aSteerRR+atan((VyCar-rCar*lWheelbase/2));
% else
%     aSlipFL=-aSteerFL+atan((VyCar+rCar*lWheelbase/2)/(VxCar-rCar*lTrackWidth/2));
%     
%     aSlipFR=-aSteerFR+atan((VyCar+rCar*lWheelbase/2)/(VxCar+rCar*lTrackWidth/2));
%     
%     aSlipRL=-aSteerRL+atan((VyCar-rCar*lWheelbase/2)/(VxCar-rCar*lTrackWidth/2));
%     
%     aSlipRR=-aSteerRR+atan((VyCar-rCar*lWheelbase/2)/(VxCar+rCar*lTrackWidth/2));
% end
% 
% end

== matlab function Simulink_Model_v12/Coef ==
  data: FzFL input; FzFR input; FzRL input; FzRR input; rSlipFL input; rSlipFR input; rSlipRL input; rSlipRR input; aSlipFL input; CoefFL output; CoefFR output; CoefRL output; CoefRR output; aSlipFR input; aSlipRL input; aSlipRR input; muTire input; KTireLong input; KTireLat input
function [CoefFL,CoefFR,CoefRL,CoefRR]...
         = Coef(FzFL,FzFR,FzRL,FzRR,...
                rSlipFL,rSlipFR,rSlipRL,rSlipRR,...
                aSlipFL,aSlipFR,aSlipRL,aSlipRR,...
                muTire,KTireLong,KTireLat)

CoefFL=muTire*FzFL*(1+rSlipFL)/(2*max(sqrt((KTireLong*rSlipFL)^2+(KTireLat*tan(aSlipFL))^2),1));

CoefFR=muTire*FzFR*(1+rSlipFR)/(2*max(sqrt((KTireLong*rSlipFR)^2+(KTireLat*tan(aSlipFR))^2),1));

CoefRL=muTire*FzRL*(1+rSlipRL)/(2*max(sqrt((KTireLong*rSlipRL)^2+(KTireLat*tan(aSlipRL))^2),1));

CoefRR=muTire*FzRR*(1+rSlipRR)/(2*max(sqrt((KTireLong*rSlipRR)^2+(KTireLat*tan(aSlipRR))^2),1));

end

== matlab function Simulink_Model_v12/axWheelCenter ==
  data: rCar input; axWheelFL output; vxCarDer input; vyCarDer input; rCarDer input; axWheelFR output; axWheelRL output; axWheelRR output; lTrackWidth input; lWheelbase input
function [axWheelFL,axWheelFR,axWheelRL,axWheelRR]...
         = axWheelCenters(rCar,vxCarDer,vyCarDer,rCarDer,...
                          lTrackWidth,lWheelbase)

axWheelFL=vxCarDer+lTrackWidth/2*rCarDer+rCar^2*lWheelbase/2;

axWheelFR=vxCarDer-lTrackWidth/2*rCarDer+rCar^2*lWheelbase/2;

axWheelRL=vxCarDer+lTrackWidth/2*rCarDer-rCar^2*lWheelbase/2;

axWheelRR=vxCarDer-lTrackWidth/2*rCarDer-rCar^2*lWheelbase/2;

end

== matlab function Simulink_Model_v12/FxTire ==
  data: rSlipFL input; FxFL output; FxFR output; FxRL output; FxRR output; rSlipFR input; rSlipRL input; rSlipRR input; fCoefFL input; fCoefFR input; fCoefRL input; fCoefRR input; muTire input; KTireLong input
function [FxFL,FxFR,FxRL,FxRR]...
         = FxTire(rSlipFL,rSlipFR,rSlipRL,rSlipRR,...
                  fCoefFL,fCoefFR,fCoefRL,fCoefRR,...
                  muTire,KTireLong)

FxFL=KTireLong*rSlipFL/(1+rSlipFL)*fCoefFL; % *((1.15-0.75*muTire)*rSlipFL^2-(1.63-0.75*muTire)*rSlipFL+1.27);

FxFR=KTireLong*rSlipFR/(1+rSlipFR)*fCoefFR; % *((1.15-0.75*muTire)*rSlipFR^2-(1.63-0.75*muTire)*rSlipFR+1.27);

FxRL=KTireLong*rSlipRL/(1+rSlipRL)*fCoefRL; % *((1.15-0.75*muTire)*rSlipRL^2-(1.63-0.75*muTire)*rSlipRL+1.27);

FxRR=KTireLong*rSlipRR/(1+rSlipRR)*fCoefRR; % *((1.15-0.75*muTire)*rSlipRR^2-(1.63-0.75*muTire)*rSlipRR+1.27);

end

== matlab function Simulink_Model_v12/FyTire ==
  data: aSlipFL input; aSlipFR input; aSlipRL input; aSlipRR input; rSlipFL input; FyFL output; FyFR output; FyRL output; FyRR output; rSlipFR input; rSlipRL input; rSlipRR input; fCoefFL input; fCoefFR input; fCoefRL input; fCoefRR input; muTire input; KTireLat input
function [FyFL,FyFR,FyRL,FyRR]...
         = FyTire(aSlipFL,aSlipFR,aSlipRL,aSlipRR,...
                  rSlipFL,rSlipFR,rSlipRL,rSlipRR,...
                  fCoefFL,fCoefFR,fCoefRL,fCoefRR,...
                  muTire,KTireLat)

FyFL=KTireLat*tan(aSlipFL)/(1+rSlipFL)*fCoefFL; % *((muTire-1.6)*tan(aSlipFL)+1.155);

FyFR=KTireLat*tan(aSlipFR)/(1+rSlipFR)*fCoefFR; % *((muTire-1.6)*tan(aSlipFR)+1.155);

FyRL=KTireLat*tan(aSlipRL)/(1+rSlipRL)*fCoefRL; % *((muTire-1.6)*tan(aSlipRL)+1.155);

FyRR=KTireLat*tan(aSlipRR)/(1+rSlipRR)*fCoefRR; % *((muTire-1.6)*tan(aSlipRR)+1.155);

end

== matlab function Simulink_Model_v12/f ==
  data: CoefFL input; fCoefFL output; CoefFR input; CoefRL input; CoefRR input; fCoefFR output; fCoefRL output; fCoefRR output
function [fCoefFL,fCoefFR,fCoefRL,fCoefRR]...
         = f(CoefFL,CoefFR,CoefRL,CoefRR)

fCoefFL=1;
if CoefFL<1
    fCoefFL=(2-CoefFL)*CoefFL;
end

fCoefFR=1;
if CoefFR<1
    fCoefFR=(2-CoefFR)*CoefFR;
end

fCoefRL=1;
if CoefRL<1
    fCoefRL=(2-CoefRL)*CoefRL;
end

fCoefRR=1;
if CoefRR<1
    fCoefRR=(2-CoefRR)*CoefRR;
end

end

== matlab function Simulink_Model_v12/rSlipDer ==
  data: nWheelFLDer input; rSlipFLDer output; nWheelFRDer input; nWheelRLDer input; nWheelRRDer input; vxWheelFL input; vxWheelFR input; vxWheelRL input; vxWheelRR input; axWheelFL input; axWheelFR input; axWheelRL input; axWheelRR input; rSlipFL input; rSlipFR input; rSlipRL input; rSlipRR input; rWheelEffective input; rSlipFRDer output; rSlipRLDer output; rSlipRRDer output
function [rSlipFLDer,rSlipFRDer,rSlipRLDer,rSlipRRDer]... 
         = rSlipDer(nWheelFLDer,nWheelFRDer,nWheelRLDer,nWheelRRDer,...
                    vxWheelFL,vxWheelFR,vxWheelRL,vxWheelRR,...
                    axWheelFL,axWheelFR,axWheelRL,axWheelRR,...
                    rSlipFL,rSlipFR,rSlipRL,rSlipRR,...
                    rWheelEffective)

if abs(vxWheelFL)<=1
    rSlipFLDer=nWheelFLDer*rWheelEffective-axWheelFL*(rSlipFL+1);
else
    rSlipFLDer=nWheelFLDer*rWheelEffective/vxWheelFL-axWheelFL/vxWheelFL^2*(rSlipFL+1);
end

if abs(vxWheelFR)<=1
    rSlipFRDer=nWheelFRDer*rWheelEffective-axWheelFR*(rSlipFR+1);
else
    rSlipFRDer=nWheelFRDer*rWheelEffective/vxWheelFR-axWheelFR/vxWheelFR^2*(rSlipFR+1);
end

if abs(vxWheelRL)<=1
    rSlipRLDer=nWheelRLDer*rWheelEffective-axWheelRL*(rSlipRL+1);
else
    rSlipRLDer=nWheelRLDer*rWheelEffective/vxWheelRL-axWheelRL/vxWheelRL^2*(rSlipRL+1);
end

if abs(vxWheelRR)<=1
    rSlipRRDer=nWheelRRDer*rWheelEffective-axWheelRR*(rSlipRR+1);
else
    rSlipRRDer=nWheelRRDer*rWheelEffective/vxWheelRR-axWheelRR/vxWheelRR^2*(rSlipRR+1);
end                
                
end

== matlab function Simulink_Model_v12/aSteering PurePursuit ==
  data: xCar input; aSteeringCmd output; yCar input; aCar input; lWheelBase input; xTrack input; yTrack input; sLookAhead input; xLookAheadPoint output; yLookAheadPoint output; NLookAheadOpt output; NLookAheadPrev input
function [aSteeringCmd,xLookAheadPoint,yLookAheadPoint,NLookAheadOpt] = aSteering(xCar,yCar,aCar,lWheelBase,xTrack,yTrack,sLookAhead,NLookAheadPrev)


NLookAheadOpt=NLookAheadPrev;
sLookAheadOpt=sqrt((xTrack(NLookAheadOpt)-xCar)^2+(yTrack(NLookAheadOpt)-yCar)^2)-sLookAhead;

for N=NLookAheadOpt+1:min(NLookAheadOpt+100,length(xTrack))
    
    NN=N %mod(N-1,length(xTrack)-1)+1;
    
    sTemp=sqrt((xTrack(NN)-xCar)^2+(yTrack(NN)-yCar)^2)-sLookAhead;
    
    if abs(sTemp)<abs(sLookAheadOpt)
        NLookAheadOpt=NN;
        sLookAheadOpt=sTemp;
    end
end

aTemp=atan2((yTrack(NLookAheadOpt)-yCar),(xTrack(NLookAheadOpt)-xCar));
aTemp=mod(aTemp+pi,2*pi)-pi;
aHeadingError=aCar-aTemp;

aSteeringCmd=-atan(2*lWheelBase*sin(aHeadingError)/sLookAhead);

xLookAheadPoint=xTrack(NLookAheadOpt);
yLookAheadPoint=yTrack(NLookAheadOpt);

%% Plot

% figure(7)
% hold on
% plot(xTrack(NLookAheadOpt),yTrack(NLookAheadOpt),'k+')
% plot(xCar,yCar,'r+')

== matlab function Simulink_Model_v12/rThrottle ==
  data: KMax output; KCurrent output; xCar input; yCar input; xTrack input; yTrack input; sAnticipation input; NClosestPointPrev input; NClosestPoint output
function [KMax,KCurrent,NClosestPoint]  = rThrottle(xCar,yCar,xTrack,yTrack,sAnticipation,NClosestPointPrev)

NClosestPoint=NClosestPointPrev;
sClosestPoint=sqrt((xTrack(NClosestPointPrev)-xCar)^2+(yTrack(NClosestPointPrev)-yCar)^2);

for N=NClosestPointPrev:NClosestPointPrev+100
    
    NN=mod(N-1,length(xTrack)-1)+1;
    
    sTemp=sqrt((xTrack(NN)-xCar)^2+(yTrack(NN)-yCar)^2);
    
    if abs(sTemp)<abs(sClosestPoint)
        NClosestPoint=NN;
        sClosestPoint=sTemp;
    end
end

%%

NTemp=max(NClosestPoint,2);
sTemp=sqrt((xTrack(NTemp)-xCar)^2+(yTrack(NTemp)-yCar)^2);

KList=zeros(1,length(xTrack));

while sTemp<sAnticipation && NTemp<length(xTrack)-1
    
    % Compute curvature
    
    A=[xTrack(NTemp-1);yTrack(NTemp-1);0];
    B=[xTrack(NTemp)  ;yTrack(NTemp)  ;0];
    C=[xTrack(NTemp+1);yTrack(NTemp+1);0];
    
    D = cross(B-A,C-A);
    b = norm(A-C);
    c = norm(A-B);
    a = norm(B-C);
    R = a*b*c/2/norm(D);
    
    K=1/R;
    KList(NTemp)=K;
    
    % Next point
    
    NTemp=NTemp+1;
    sTemp=sTemp+sqrt((xTrack(NTemp)-xTrack(NTemp-1))^2+(yTrack(NTemp)-yTrack(NTemp-1))^2);
end
    
KTemp=maxk(KList,min(3,length(KList)));
KMax=KTemp(min(3,length(KList)));
KCurrent=KList(1);

== matlab function Simulink_Model_v12/NLap ==
  data: xCar input; BNewLap output; yCar input; xCarPrev input; yCarPrev input; xStartLine input; yStartLine input
function BNewLap ...
         = NLap(xCar,yCar,...
                xCarPrev,yCarPrev,...
                xStartLine,yStartLine)
BNewLap=0;
            
if xCar==xCarPrev && yCar==yCarPrev
    BNewLap=0;
end

% https://ericleong.me/research/circle-line/

x1=xCar;            y1=yCar;
x2=xCarPrev;        y2=yCarPrev;
x3=xStartLine(1);   y3=yStartLine(1);
x4=xStartLine(2);   y4=yStartLine(2);


a1=y2-y1;           a2=y4-y3;
b1=x1-x2;           b2=x3-x4;
c1=a1*x1+b1*y1;     c2=a2*x3+b2*y3;

d=det([a1,b1;a2,b2]);

if d==0
    BNewLap=0
end

x=det([c1,b1;c2,b2])/d;
y=det([a1,c1;a2,c2])/d;

if x >= min(x1, x2) && x <= max(x1, x2) ...
   && x >= min(x3, x4) && x <= max(x3, x4) ...
   && y >= min(y1, y2) && y <= max(y1, y2) ...
   && y >= min(y3, y4) && y <= max(y3, y4)

    BNewLap=1;
end

end

== matlab function Simulink_Model_v12/sStep ==
  data: xCar input; sStep output; yCar input; xCarPrev input; yCarPrev input
function sStep ...
         = sStep(xCar,yCar,...
                xCarPrev,yCarPrev)

sStep=sqrt((xCar-xCarPrev)^2+(yCar-yCarPrev)^2)

end

== stateflow chart Simulink_Model_v12/Chart ==
  state Gear1
    en:
    Gear=1;
  state Gear2
    en:
    Gear=2;
  (default) -> Gear1
  Gear1 -> Gear2 : [vCar>9.5]
  Gear2 -> Gear1 : [vCar<9]
  data: vCar input; Gear output

== matlab function Simulink_Model_v12/NClosestPoint ==
  data: xCar input; NClosestPoint output; yCar input; xTrack input; yTrack input; NClosestPointPrev input
function NClosestPoint   = NClosestPoint(xCar,yCar,xTrack,yTrack,NClosestPointPrev)


NClosestPoint=NClosestPointPrev;
sClosestPoint=sqrt((xTrack(NClosestPointPrev)-xCar)^2+(yTrack(NClosestPointPrev)-yCar)^2);

for N=NClosestPointPrev:NClosestPointPrev+100
    
    NN=mod(N-1,length(xTrack))+1;
    
    sTemp=sqrt((xTrack(NN)-xCar)^2+(yTrack(NN)-yCar)^2);
    
    if abs(sTemp)<abs(sClosestPoint)
        NClosestPoint=NN;
        sClosestPoint=sTemp;
    end
end

% NClosestPoint=NClosestPoint+1;
% sClosestPoint=sqrt((xTrack(NClosestPoint)-xCar)^2+(yTrack(NClosestPoint)-yCar)^2);

== matlab function Simulink_Model_v12/Trajectory ==
  data: BOpt input; xCar input; yCar input; xTrack input; yTrack input; lHalfTrackWidth input; NClosestPoint input; xTraj output; yTraj output; rTrajOpt input
function [xTraj,yTraj]   = Trajectory(BOpt,xCar,yCar,xTrack,yTrack,lHalfTrackWidth,NClosestPoint,rTrajOpt)

% plot(xTrack(NClosestPoint),yTrack(NClosestPoint),'r+')

NAnticipation=100;

% xTrack=[xTrack(NClosestPoint:end),xTrack(1:NClosestPoint-1)]
% yTrack=[yTrack(NClosestPoint:end),yTrack(1:NClosestPoint-1)]


xTemp=zeros(1,length(xTrack));
yTemp=zeros(1,length(yTrack));

for i=1:length(xTrack)
    
    II=mod(i+NClosestPoint-2,length(xTrack))+1;
    
    xTemp(i)=xTrack(II);
    yTemp(i)=yTrack(II);
end

xTrack=xTemp;
yTrack=yTemp;
    
%% Track Sides

X=[xTrack(end),xTrack(1:NAnticipation+1)];
Y=[yTrack(end),yTrack(1:NAnticipation+1)];

B=[0;0;1];

xyRightSide=zeros(3,NAnticipation);
xyLeftSide =zeros(3,NAnticipation);

for i=2:NAnticipation+1

    A=[X(i+1)-X(i-1);Y(i+1)-Y(i-1);0];

    R=cross(A,B);
    L=cross(A,-B);

    xyRightSide(:,i-1)=lHalfTrackWidth*R/norm(R)+[X(i);Y(i);0];
    xyLeftSide (:,i-1)=lHalfTrackWidth*L/norm(L)+[X(i);Y(i);0];

end

%% Shortest trajectory

H_S=zeros(NAnticipation,NAnticipation);

B_S=zeros(1,NAnticipation);

for i=1:NAnticipation-1

    % H
    dx  =(xyLeftSide(1,i)  -xyRightSide(1,i)  );
    dxp1=(xyLeftSide(1,i+1)-xyRightSide(1,i+1));

    h_x=[dx^2,-dx*dxp1;...
         -dx*dxp1,dxp1^2];

    dy  =(xyLeftSide(2,i)  -xyRightSide(2,i)  );
    dyp1=(xyLeftSide(2,i+1)-xyRightSide(2,i+1));

    h_y=[dy^2,-dy*dyp1;...
         -dy*dyp1,dyp1^2];

    H_S(i:i+1,i:i+1)=H_S(i:i+1,i:i+1)+h_x+h_y;

    % B
    b_x=2*(xyRightSide(1,i+1)-xyRightSide(1,i))*[-dx,dxp1];

    b_y=2*(xyRightSide(2,i+1)-xyRightSide(2,i))*[-dy,dyp1];

    B_S(i:i+1)=B_S(i:i+1)+b_x+b_y;
end

%% Minimum Curvature

H_C=zeros(NAnticipation,NAnticipation);

B_C=zeros(1,NAnticipation);

for i=2:NAnticipation-1

    % H
    dxm1=(xyLeftSide(1,i-1)-xyRightSide(1,i-1))
    dx  =(xyLeftSide(1,i)  -xyRightSide(1,i)  );
    dxp1=(xyLeftSide(1,i+1)-xyRightSide(1,i+1));

    h_x=[dxm1^2, -2*dxm1*dx, dxm1*dxp1;...
         -2*dx*dxm1, 4*dx^2, -2*dx*dxp1;...
         dxp1*dxm1, -2*dxp1*dx,dxp1^2];

    dym1=(xyLeftSide(2,i-1)-xyRightSide(2,i-1));
    dy  =(xyLeftSide(2,i)  -xyRightSide(2,i)  );
    dyp1=(xyLeftSide(2,i+1)-xyRightSide(2,i+1));

    h_y=[dym1^2, -2*dym1*dy, dym1*dyp1;...
         -2*dy*dym1, 4*dy^2, -2*dy*dyp1;...
         dyp1*dym1, -2*dyp1*dy,dyp1^2];

    H_C(i-1:i+1,i-1:i+1)=H_C(i-1:i+1,i-1:i+1)+h_x+h_y;

    % B
    b_x=2*(xyRightSide(1,i+1)-2*xyRightSide(1,i)+xyRightSide(1,i-1))*[dxm1, -2*dx, dxp1];

    b_y=2*(xyRightSide(2,i+1)-2*xyRightSide(2,i)+xyRightSide(2,i-1))*[dym1, -2*dy, dyp1];

    B_C(i-1:i+1)=B_C(i-1:i+1)+b_x+b_y;
end

%% Problem Formulation

H=rTrajOpt*H_S/norm(H_S)+(1-rTrajOpt)*H_C/norm(H_C);

B=rTrajOpt*B_S/norm(H_S)+(1-rTrajOpt)*B_C/norm(H_C);

%% Find current alpha
% https://fr.mathworks.com/matlabcentral/answers/26464-projecting-a-point-onto-a-line

p0=xyRightSide(1:2,1);
p1=xyLeftSide(1:2,1);
q=[xCar;yCar];

a = [-q(1)*(p1(1)-p0(1)) - q(2)*(p1(2)-p0(2)); ...
    -p0(2)*(p1(1)-p0(1)) + p0(1)*(p1(2)-p0(2))]; 
b = [p1(1) - p0(1), p1(2) - p0(2);...
    p0(2) - p1(2), p1(1) - p0(1)];
c = -(b\a);

alpha_0=norm(c-p0)/(2*lHalfTrackWidth)
if norm(c-p1)>(2*lHalfTrackWidth) && norm(c-p1)>norm(c-p0)
    alpha_0=0;
end
alpha_0=max(min(alpha_0,0.9),0.1)

%% quadprog

A=[eye(NAnticipation);-eye(NAnticipation)];
b=[0.95*ones(NAnticipation,1);-0.05*ones(NAnticipation,1)];

Aeq=zeros(NAnticipation,NAnticipation);
Aeq(1,1)=1;
% Aeq(2,2)=1;
beq=[alpha_0;zeros(NAnticipation-1,1)];

lb=zeros(NAnticipation,1);
ub=ones(NAnticipation,1);
x0=0.5*ones(NAnticipation,1);

coder.extrinsic('quadprog');
options=optimset('Display', 'off'); 
% options=optimoptions('quadprog','Algorithm','active-set');
alpha=0.5*ones(NAnticipation,1);

if BOpt
    alpha=quadprog(2*H,B',A,b,Aeq,beq,lb,ub,x0,options); % isfinite ?
end

%% Solution handling

xTraj=zeros(1,NAnticipation);
yTraj=zeros(1,NAnticipation);

for i=1:NAnticipation

    xTraj(i)=xyRightSide(1,i)+alpha(i)*(xyLeftSide(1,i)-xyRightSide(1,i))
    yTraj(i)=xyRightSide(2,i)+alpha(i)*(xyLeftSide(2,i)-xyRightSide(2,i))
    
end

%% Plot 

% figure(7)
% hold on
% plot(xTraj(1),yTraj(1),'k+')
% plot(xCar,yCar,'r+')

== matlab function Simulink_Model_v12/vxWheelCenter ==
  data: vxWheelFL output; vxCar input; vyCar input; rCar input; vxWheelFR output; vxWheelRL output; vxWheelRR output; lTrackWidth input
function [vxWheelFL,vxWheelFR,vxWheelRL,vxWheelRR]...
         = vxWheelCenters(vxCar,vyCar,rCar,...
                          lTrackWidth)

vxWheelFL=vxCar+lTrackWidth/2*rCar;

vxWheelFR=vxCar-lTrackWidth/2*rCar;

vxWheelRL=vxCar+lTrackWidth/2*rCar;

vxWheelRR=vxCar-lTrackWidth/2*rCar;

end

== matlab function Simulink_Model_v12/FMCar ==
  data: FxFL input; FxCar output; FxFR input; FxRL input; FxRR input; FyFL input; FyFR input; FyRL input; FyRR input; aSteerFL input; aSteerFR input; aSteerRL input; aSteerRR input; lTrackWidth input; lWheelbase input; FyCar output; MzCar output
function [FxCar,FyCar,MzCar]...
         = FMCar(FxFL,FxFR,FxRL,FxRR,...
                 FyFL,FyFR,FyRL,FyRR,...
                 aSteerFL,aSteerFR,aSteerRL,aSteerRR,...
                 lTrackWidth,lWheelbase)

FxCar=FxFL*cos(aSteerFL)-FyFL*sin(aSteerFL)+FxFR*cos(aSteerFR)-FyFR*sin(aSteerFR)...
      +FxRL*cos(aSteerRL)-FyRL*sin(aSteerRL)+FxRR*cos(aSteerRR)-FyRR*sin(aSteerRR);

FyCar=FxFL*sin(aSteerFL)+FyFL*cos(aSteerFL)+FxFR*sin(aSteerFR)+FyFR*cos(aSteerFR)...
      +FxRL*sin(aSteerRL)+FyRL*cos(aSteerRL)+FxRR*sin(aSteerRR)+FyRR*cos(aSteerRR);

MzCar=lTrackWidth/2*(-FxFL*cos(aSteerFL)+FyFL*sin(aSteerFL)-FxRL*cos(aSteerRL)+FyRL*sin(aSteerRL))...
      +lTrackWidth/2*(FxFR*cos(aSteerFR)-FyFR*sin(aSteerFR)+FxRR*cos(aSteerRR)-FyRR*sin(aSteerRR))...
      +lWheelbase/2*(FxFL*sin(aSteerFL)+FyFL*cos(aSteerFL)+FxFR*sin(aSteerFR)+FyFR*cos(aSteerFR))...
      +lWheelbase/2*(-FxRL*sin(aSteerRL)-FyRL*cos(aSteerRL)-FxRR*sin(aSteerRR)-FyRR*cos(aSteerRR));

end
